simulink model "State_Flow_D"  (R2017a)
settings: Solver=FixedStepDiscrete  StartTime=0.0  StopTime=inf  FixedStep=0.001  RelTol=1e-3  EnableMultiTasking=on
libraries: xpcethercatlib x35, simulink x11, commutil2 x2
(part 1 of 3)
settings Model: SimulationMode=external  Creator=simoc  LastModifiedBy=Danie
settings SolverCC: EnableConcurrentExecution=on  ConcurrentTasks=on  AutoInsertRateTranBlk=on
settings DataIOCC: SaveFormat=StructureWithTime
settings OptimizationCC: BlockReduction=off  OptimizeBlockIOStorage=off  BufferReuse=off  GlobalBufferReuse=off  ExpressionFolding=off  LocalBlockOutputs=off
settings HardwareCC: ProdBitPerPointer=32  ProdBitPerSizeT=32  ProdBitPerPtrDiffT=32  ProdLargestAtomicFloat=None  ProdWordSize=32  ProdLongLongMode=on  ProdHWDeviceType=Generic->32-bit x86 compatible
settings RTWCC: SystemTargetFile=slrt.tlc  TemplateMakefile=slrt_default_tmf  Description=Simulink Real-Time  RTWCompilerOptimization=on
settings SimulinkRealTimeCC: xPCConcurrentTasks=on

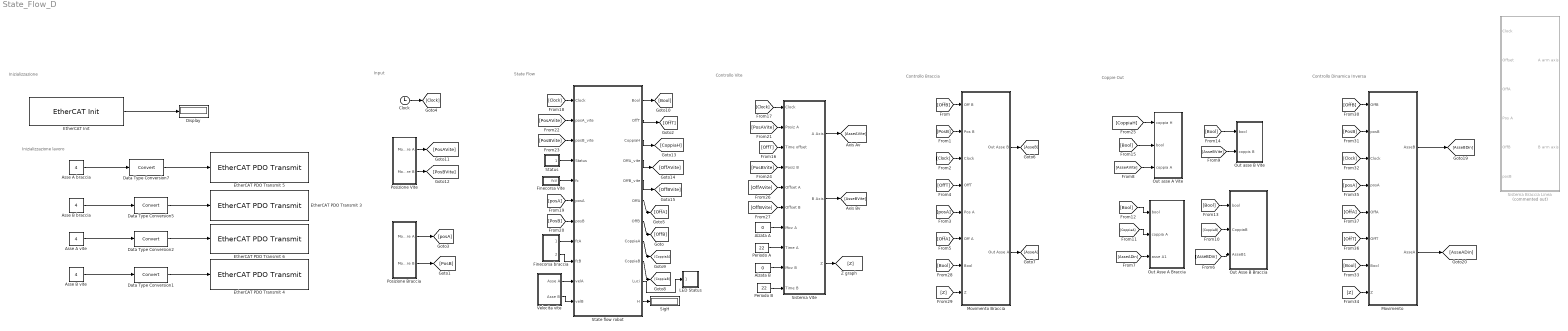
== system State_Flow_D ==
  note: Input
  note: State Flow
  note: Coppie Out
  note: Controllo Braccia
  note: Controllo Vite
  note: Inizializzazione
  note: Inizializzazione lavoro
  note: Controllo Dinamica Inversa
  Alzata A : Constant  Value=0
  "Alzata B " : Constant  Value=0
  Asse A braccia : Constant  Value=4
  Asse A vite : Constant  Value=4
  Asse B braccia : Constant  Value=4
  Asse B vite : Constant  Value=4
  Clock : Clock
  Data Type Conversion{1..2,5,7} (4 alike) : DataTypeConversion
  Display : Display
  "EtherCAT Init " : xpcethercatlib/EtherCAT Init   Priority=0  config_file=C:\Users\Danie\Documenti\Github\PKMRobot\final_net.xml  device_id=0  pci_bus=4  pci_slot=1  dctuning=0  enaDebug=off  enaDC=on  errLink=off  masterDbg=off  stateChgDbg=off  baseClock=off  masterCfg=off  logFile='c:\dbglog.txt'  sample_time=0.001000  DCMode=1
      settings: SourceProductName=Simulink Real-Time  SourceProductBaseCode=XP
  EtherCAT PDO Transmit 3 : xpcethercatlib/EtherCAT PDO Transmit   Priority=3  sig_name=AZ2.Receive PDO 1.Axis A Modes of operation  sig_offset=264  sig_type=int8  type_size=8  sig_dim=1  device_id=0  sample_time=0.001000
      settings: SourceProductName=Simulink Real-Time  SourceProductBaseCode=XP
  EtherCAT PDO Transmit 4 : xpcethercatlib/EtherCAT PDO Transmit   Priority=3  sig_name=AZ2.Receive PDO 1.Axis A Modes of operation  sig_offset=264  sig_type=int8  type_size=8  sig_dim=1  device_id=0  sample_time=0.001000
      settings: SourceProductName=Simulink Real-Time  SourceProductBaseCode=XP
  EtherCAT PDO Transmit 5 : xpcethercatlib/EtherCAT PDO Transmit   Priority=3  sig_name=AZ2.Receive PDO 2.Axis B Modes of operation  sig_offset=288  sig_type=int8  type_size=8  sig_dim=1  device_id=0  sample_time=0.001000
      settings: SourceProductName=Simulink Real-Time  SourceProductBaseCode=XP
  EtherCAT PDO Transmit 6 : xpcethercatlib/EtherCAT PDO Transmit   Priority=3  sig_name=AZ2.Receive PDO 1.Axis A Modes of operation  sig_offset=264  sig_type=int8  type_size=8  sig_dim=1  device_id=0  sample_time=0.001000
      settings: SourceProductName=Simulink Real-Time  SourceProductBaseCode=XP
  Finecorsa Vite : Subsystem
  Finecorsa braccia : Subsystem
  LED Status : Subsystem
  Movimento : Subsystem
  Movimento Braccia : Subsystem
  Out Asse A Braccia : Subsystem
  Out Asse B Braccia : Subsystem
  Out asse A Vite : Subsystem
  Out asse B Vite : Subsystem
  Periodo A : Constant  Value=22
  Periodo B : Constant  Value=22
  "Posizione Braccia " : Subsystem
  Posizione Vite : Subsystem
  SigH : Display
  Sistema Braccia Linea : Subsystem  Commented=on
  Sistema Vite : Subsystem
  State flow robot : Stateflow chart  TreatAsAtomicUnit=on
  Status : Subsystem
  "Velocita vite " : Subsystem
  wires:
  "EtherCAT Init "/1 -> Display/1
  Data Type Conversion7/1 -> EtherCAT PDO Transmit 5/1
  Asse A braccia/1 -> Data Type Conversion7/1
  Data Type Conversion5/1 -> EtherCAT PDO Transmit 3/1
  Asse B braccia/1 -> Data Type Conversion5/1
  Clock/1 -> [Clock]
  State flow robot/1(Bool) -> [Bool]
  Data Type Conversion1/1 -> EtherCAT PDO Transmit 4/1
  Asse B vite/1 -> Data Type Conversion1/1
  Data Type Conversion2/1 -> EtherCAT PDO Transmit 6/1
  Asse A vite/1 -> Data Type Conversion2/1
  Posizione Vite/2(Motore B) -> [PosBVite]
  Status/1(Word) -> State flow robot/4(Status)
  State flow robot/2(OffT) -> [OffT]
  Alzata A/1 -> Sistema Vite/7(Mov A)
  Periodo A/1 -> Sistema Vite/8(Time A)
  "Alzata B "/1 -> Sistema Vite/9(Mov B)
  Periodo B/1 -> Sistema Vite/10(Time B)
  Finecorsa Vite/1(fcV) -> State flow robot/5(fc)
  Finecorsa braccia/1(Asse A) -> State flow robot/8(fcA)
  Finecorsa braccia/2(Asse B) -> State flow robot/9(fcB)
  "Posizione Braccia "/2(Motore B) -> [PosB]
  "Posizione Braccia "/1(Motore A) -> [posA]
  Posizione Vite/1(Motore A) -> [PosAVite]
  State flow robot/10(Luci) -> LED Status/1(Luci)
  "Velocita vite "/1(Asse A) -> State flow robot/10(velA)
  "Velocita vite "/2(Asse B) -> State flow robot/11(velB)
  State flow robot/7(OffB) -> [OffB]
  State flow robot/6(OffA) -> [OffA]
  [AsseBDin] -> Out Asse B Braccia/3(AsseB1)
  [AsseADin] -> Out Asse A Braccia/3(asse A1)
  [CoppiaB] -> Out Asse B Braccia/2(CoppiaB)
  State flow robot/9(CoppiaB) -> [CoppiaB]
  State flow robot/8(CoppiaA) -> [CoppiaA]
  [CoppiaA] -> Out Asse A Braccia/2(coppia A)
  [Bool] -> Out Asse A Braccia/1(bool)
  [Bool] -> Out Asse B Braccia/1(bool)
  [Bool] -> Out asse B Vite/1(bool)
  [Bool] -> Out asse A Vite/2(bool)
  [OffT] -> Sistema Vite/3(Time offset)
  [Clock] -> Sistema Vite/1(Clock)
  [Clock] -> State flow robot/1(Clock)
  [posA] -> State flow robot/6(posA)
  [PosB] -> State flow robot/7(posB)
  [PosAVite] -> Sistema Vite/2(Posiz A)
  [PosAVite] -> State flow robot/2(posA_vite)
  [PosBVite] -> State flow robot/3(posB_vite)
  [PosBVite] -> Sistema Vite/4(Posiz B)
  State flow robot/3(CoppiaH) -> [CoppiaH]
  [CoppiaH] -> Out asse A Vite/1(coppia H)
  State flow robot/4(OffA_vite) -> [OffAVite]
  [OffAVite] -> Sistema Vite/5(Offset A)
  State flow robot/5(OffB_vite) -> [OffBVite]
  [OffBVite] -> Sistema Vite/6(Offset B)
  [OffB] -> Movimento Braccia/1(Off B)
  [PosB] -> Movimento Braccia/2(Pos B)
  [Clock] -> Movimento Braccia/3(Clock)
  [OffT] -> Movimento Braccia/4(OffT)
  [posA] -> Movimento Braccia/5(Pos A)
  [OffA] -> Movimento Braccia/6(Off A)
  Movimento Braccia/1(Out Asse B) -> [AsseB]
  Movimento Braccia/2(Out Asse A) -> [AsseA]
  Sistema Vite/1(A Axis) -> [AsseAVite]
  [AsseAVite] -> Out asse A Vite/3(coppia A)
  Sistema Vite/2(B Axis) -> [AsseBVite]
  [AsseBVite] -> Out asse B Vite/2(coppis B)
  [Bool] -> Movimento Braccia/7("Bool ")
  Sistema Vite/3(Z) -> [Z]
  [Z] -> Movimento Braccia/8(Z)
  [PosB] -> Movimento/2(posB)
  Movimento/2(AsseA) -> [AsseADin]
  Movimento/1(AsseB) -> [AsseBDin]
  [OffA] -> Movimento/5(OffA)
  [OffT] -> Movimento/6(OffT)
  [OffB] -> Movimento/1(OffB)
  [Clock] -> Movimento/3(Clock)
  [posA] -> Movimento/4(posA)
  [Bool] -> Movimento/7("Bool ")
  [Z] -> Movimento/8(Z)
  State flow robot/11(H) -> SigH/1

== system State_Flow_D/Finecorsa Vite ==
  Data Type Conversion8 : DataTypeConversion
  EtherCAT PDO Receive16 : xpcethercatlib/EtherCAT PDO Receive  Priority=2  sig_name=AZ2.Transmit PDO 3.General purpose inputs  sig_offset=440  sig_type=uint16  type_size=16  sig_dim=1  device_id=0  sample_time=0.001000
      settings: SourceProductName=Simulink Real-Time  SourceProductBaseCode=XP
  Integer to Bit Converter : commutil2/Integer to Bit Converter  nbits=16  signedInputValues=Unsigned  bitOrder=LSB first  outDtype=Inherit via internal rule
  Selector : Selector  InputPortWidth=16  IndexOptions=Index vector (dialog)  Indices=15  OutputSizes=1
  fcV : Outport
  wires:
  EtherCAT PDO Receive16/1 -> Data Type Conversion8/1
  Selector/1 -> fcV/1
  Data Type Conversion8/1 -> Integer to Bit Converter/1
  Integer to Bit Converter/1 -> Selector/1

== system State_Flow_D/Finecorsa braccia ==
  Data Type Conversion8 : DataTypeConversion
  EtherCAT PDO Receive16 : xpcethercatlib/EtherCAT PDO Receive  Priority=2  sig_name=AZ1.Transmit PDO 3.General purpose inputs  sig_offset=184  sig_type=uint16  type_size=16  sig_dim=1  device_id=0  sample_time=0.001000
      settings: SourceProductName=Simulink Real-Time  SourceProductBaseCode=XP
  Integer to Bit Converter : commutil2/Integer to Bit Converter  nbits=16  signedInputValues=Unsigned  bitOrder=LSB first  outDtype=Inherit via internal rule
  Selector : Selector  InputPortWidth=16  IndexOptions=Index vector (dialog)  Indices=8  OutputSizes=1
  Selector1 : Selector  InputPortWidth=16  IndexOptions=Index vector (dialog)  Indices=15  OutputSizes=1
  Asse A : Outport
  Asse B : Outport  Port=2
  wires:
  Data Type Conversion8/1 -> Integer to Bit Converter/1
  Integer to Bit Converter/1 -> Selector1/1, Selector/1
  EtherCAT PDO Receive16/1 -> Data Type Conversion8/1
  Selector1/1 -> Asse B/1
  Selector/1 -> Asse A/1

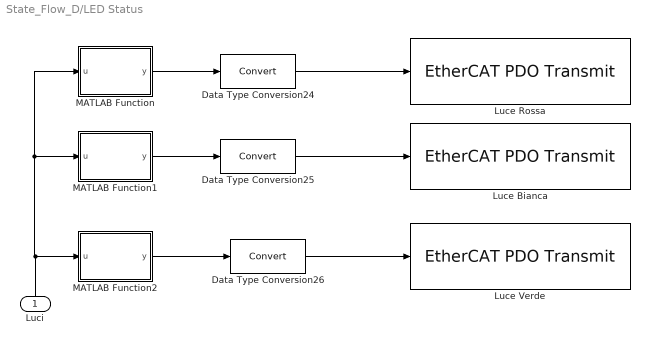
== system State_Flow_D/LED Status ==
  Luci : Inport
  Data Type Conversion24 : DataTypeConversion
  Data Type Conversion25 : DataTypeConversion
  Data Type Conversion26 : DataTypeConversion
  Luce Bianca : xpcethercatlib/EtherCAT PDO Transmit   Priority=3  sig_name=Beckoff.Channel 6.Output  sig_offset=1  sig_type=boolean  type_size=1  sig_dim=1  device_id=0  sample_time=0.001000
      settings: SourceProductName=Simulink Real-Time  SourceProductBaseCode=XP
  "Luce Rossa " : xpcethercatlib/EtherCAT PDO Transmit   Priority=3  sig_name=Beckoff.Channel 8.Output  sig_offset=3  sig_type=boolean  type_size=1  sig_dim=1  device_id=0  sample_time=0.001000
      settings: SourceProductName=Simulink Real-Time  SourceProductBaseCode=XP
  Luce Verde : xpcethercatlib/EtherCAT PDO Transmit   Priority=3  sig_name=Beckoff.Channel 7.Output  sig_offset=2  sig_type=boolean  type_size=1  sig_dim=1  device_id=0  sample_time=0.001000
      settings: SourceProductName=Simulink Real-Time  SourceProductBaseCode=XP
  MATLAB Function : MATLAB Function  TreatAsAtomicUnit=on
  MATLAB Function1 : MATLAB Function  TreatAsAtomicUnit=on
  MATLAB Function2 : MATLAB Function  TreatAsAtomicUnit=on
  wires:
  MATLAB Function2/1(y) -> Data Type Conversion26/1
  MATLAB Function/1(y) -> Data Type Conversion24/1
  Data Type Conversion26/1 -> Luce Verde/1
  MATLAB Function1/1(y) -> Data Type Conversion25/1
  Data Type Conversion24/1 -> "Luce Rossa "/1
  Data Type Conversion25/1 -> Luce Bianca/1
  Luci/1 -> MATLAB Function/1(u), MATLAB Function1/1(u), MATLAB Function2/1(u)

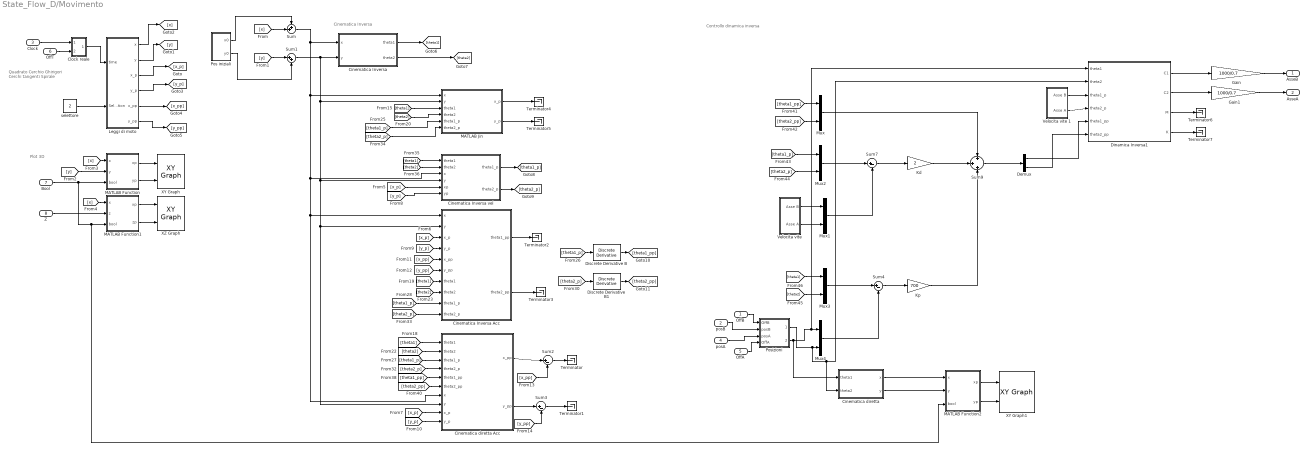
== system State_Flow_D/Movimento ==
  note: Cinematica Inversa
  note: Controllo dinamica inversa
  note: Plot 3D
  note: Quadrato
      | Cerchio
      | Ghirigori
      | Cerchi tangenti
      | Spirale
  OffB : Inport
  posB : Inport  Port=2
  Clock : Inport  Port=3
  posA : Inport  Port=4
  OffA : Inport  Port=5
  OffT : Inport  Port=6
  "Bool " : Inport  Port=7
  Z : Inport  Port=8
  Cinematica Inversa : MATLAB Function  TreatAsAtomicUnit=on
  Cinematica Inversa Acc : MATLAB Function  TreatAsAtomicUnit=on
  Cinematica Inversa vel : MATLAB Function  TreatAsAtomicUnit=on
  Cinematica diretta : MATLAB Function  TreatAsAtomicUnit=on
  Cinematica diretta Acc : MATLAB Function  TreatAsAtomicUnit=on
  Clock reale : Subsystem
  Demux : Demux  Outputs=2
  Dinamica Inversa1 : MATLAB Function  TreatAsAtomicUnit=on
  Discrete Derivative B : simulink/Discrete/Discrete Derivative  gainval=1.0  ICPrevScaledInput=0.0  OutMin=[]  OutMax=[]  OutDataType=fixdt(1, 16)  OutScaling=2^-10  DoSatur=off
  Discrete Derivative B1 : simulink/Discrete/Discrete Derivative  gainval=1.0  ICPrevScaledInput=0.0  OutMin=[]  OutMax=[]  OutDataType=fixdt(1, 16)  OutScaling=2^-10  DoSatur=off
  Gain : Gain  Gain=1000/0.7
  Gain1 : Gain  Gain=1000/0.7
  Kd : Gain  Gain=2
  Kp : Gain  Gain=700
  Leggi di moto : Subsystem
  MATLAB Function : MATLAB Function  TreatAsAtomicUnit=on
  MATLAB Function1 : MATLAB Function  TreatAsAtomicUnit=on
  MATLAB Function2 : MATLAB Function  TreatAsAtomicUnit=on
  MATLAB Jin : MATLAB Function  TreatAsAtomicUnit=on
  Mux{,1..4} (5 alike) : Mux  Inputs=2
  Pos iniziali : Subsystem
  Posizioni : Subsystem
  Sum : Sum  Inputs=++|
  Sum1 : Sum  Inputs=|++
  Sum{2..4,7} (4 alike) : Sum  Inputs=|+-
  Sum9 : Sum  Inputs=+|+|+
  Terminator{,1..7} (8 alike) : Terminator
  "Velocita vite " : Subsystem
  Velocita vite 1 : Subsystem
  XY Graph : simulink/Sinks/XY Graph  xmin=-0.1  xmax=0.1  ymin=-0.1  ymax=0.1  st=0.001
  XY Graph1 : simulink/Sinks/XY Graph  xmin=-0.15  xmax=0.15  ymin=0  ymax=0.5  st=0.001
  XZ Graph : simulink/Sinks/XY Graph  xmin=-0.15  xmax=0.15  ymin=-0.15  ymax=0.15  st=0.001
  selettore : Constant  Value=2
  AsseB : Outport
  AsseA : Outport  Port=2
  wires:
  Sum/1 -> Cinematica diretta Acc/7(x), Cinematica Inversa Acc/1(x), Cinematica Inversa vel/3(x), MATLAB Jin/1(x), Cinematica Inversa/1(x)
  Clock/1 -> Clock reale/1(cr)
  OffT/1 -> Clock reale/2(offset)
  Cinematica diretta Acc/1(x_pp) -> Sum2/1
  Cinematica diretta Acc/2(y_pp) -> Sum3/1
  Sum2/1 -> Terminator/1
  Sum3/1 -> Terminator1/1
  MATLAB Jin/1(x_p) -> Terminator4/1
  MATLAB Jin/2(y_p) -> Terminator5/1
  Sum1/1 -> Cinematica diretta Acc/8(y), Cinematica Inversa Acc/2(y), Cinematica Inversa vel/4(y), MATLAB Jin/2(y), Cinematica Inversa/2(y)
  Clock reale/1(Ck) -> Leggi di moto/1(time)
  Leggi di moto/2(y) -> [y]
  [x] -> MATLAB Function1/1(x)
  [x] -> MATLAB Function/1(x)
  Leggi di moto/1(x) -> [x]
  Leggi di moto/3(x_p) -> [x_p]
  [y] -> MATLAB Function/2(y)
  selettore/1 -> Leggi di moto/2(Selection)
  MATLAB Function/1(xp) -> XY Graph/1
  MATLAB Function1/1(xp) -> XZ Graph/1
  Z/1 -> MATLAB Function1/2(z)
  Leggi di moto/4(y_p) -> [y_p]
  MATLAB Function1/2(zp) -> XZ Graph/2
  MATLAB Function/2(yp) -> XY Graph/2
  [y] -> Sum1/1
  Leggi di moto/5(x_pp) -> [x_pp]
  Leggi di moto/6(y_pp) -> [y_pp]
  [x_p] -> Cinematica Inversa vel/5(xp)
  [x_p] -> Cinematica Inversa Acc/3(x_p)
  [x_p] -> Cinematica diretta Acc/9(x_p)
  [y_p] -> Cinematica Inversa vel/6(yp)
  [y_p] -> Cinematica Inversa Acc/4(y_p)
  [y_p] -> Cinematica diretta Acc/10(y_p)
  [x_pp] -> Cinematica Inversa Acc/5(x_pp)
  [y_pp] -> Cinematica Inversa Acc/6(y_pp)
  [x_pp] -> Sum2/2
  [y_pp] -> Sum3/2
  Cinematica Inversa Acc/1(theta1_pp) -> Terminator2/1
  Cinematica Inversa Acc/2(theta2_pp) -> Terminator3/1
  OffB/1 -> Posizioni/1(OffB)
  posB/1 -> Posizioni/2(posB)
  posA/1 -> Posizioni/3(posA)
  OffA/1 -> Posizioni/4(OffA)
  Cinematica Inversa/1(theta1) -> [theta1]
  [theta1] -> MATLAB Jin/3(theta1)
  [theta1] -> Cinematica diretta Acc/1(theta1)
  [theta1] -> Cinematica Inversa Acc/7(theta1)
  Cinematica Inversa/2(theta2) -> [theta2]
  [theta2] -> MATLAB Jin/4(theta2)
  [theta2] -> Cinematica diretta Acc/2(theta2)
  [theta2] -> Cinematica Inversa Acc/8(theta2)
  Cinematica Inversa vel/1(theta1_p) -> [theta1_p]
  [theta1_p] -> MATLAB Jin/5(theta1_p)
  [theta1_p] -> Discrete Derivative B/1
  [theta1_p] -> Cinematica diretta Acc/3(theta1_p)
  [theta1_p] -> Cinematica Inversa Acc/9(theta1_p)
  Cinematica Inversa vel/2(theta2_p) -> [theta2_p]
  [theta2_p] -> Discrete Derivative B1/1
  [theta2_p] -> Cinematica diretta Acc/4(theta2_p)
  [theta2_p] -> Cinematica Inversa Acc/10(theta2_p)
  [theta2_p] -> MATLAB Jin/6(theta2_p)
  [theta1] -> Cinematica Inversa vel/1(theta1)
  [theta2] -> Cinematica Inversa vel/2(theta2)
  Discrete Derivative B/1 -> [theta1_pp]
  [theta1_pp] -> Cinematica diretta Acc/5(theta1_pp)
  Discrete Derivative B1/1 -> [theta2_pp]
  [theta2_pp] -> Cinematica diretta Acc/6(theta2_pp)
  Pos iniziali/2(y0) -> Sum1/2
  [x] -> Sum/2
  Pos iniziali/1(x0) -> Sum/1
  [theta1_pp] -> Mux/1
  [theta2_pp] -> Mux/2
  "Velocita vite "/2(Asse A) -> Mux1/2
  "Velocita vite "/1(Asse B) -> Mux1/1
  [theta1_p] -> Mux2/1
  [theta2_p] -> Mux2/2
  [theta1] -> Mux3/1
  [theta2] -> Mux3/2
  Mux2/1 -> Sum7/1
  Mux1/1 -> Sum7/2
  Mux3/1 -> Sum4/1
  Mux4/1 -> Sum4/2
  Mux/1 -> Sum9/1
  Sum7/1 -> Kd/1
  Sum4/1 -> Kp/1
  Kp/1 -> Sum9/3
  Kd/1 -> Sum9/2
  Sum9/1 -> Demux/1
  Velocita vite 1/2(Asse A) -> Dinamica Inversa1/4(theta2_p)
  Velocita vite 1/1(Asse B) -> Dinamica Inversa1/3(theta1_p)
  Posizioni/2(Asse Bb) -> Cinematica diretta/1(theta1), Dinamica Inversa1/1(theta1), Mux4/1
  Posizioni/1(Asse Ab) -> Cinematica diretta/2(theta2), Dinamica Inversa1/2(theta2), Mux4/2
  Demux/1 -> Dinamica Inversa1/5(theta1_pp)
  Demux/2 -> Dinamica Inversa1/6(theta2_pp)
  Dinamica Inversa1/1(C1) -> Gain/1
  Dinamica Inversa1/2(C2) -> Gain1/1
  Gain/1 -> AsseB/1
  Gain1/1 -> AsseA/1
  MATLAB Function2/1(xp) -> XY Graph1/1
  MATLAB Function2/2(yp) -> XY Graph1/2
  "Bool "/1 -> MATLAB Function2/3(bool), MATLAB Function1/3(bool), MATLAB Function/3(bool)
  Cinematica diretta/2(y) -> MATLAB Function2/2(y)
  Cinematica diretta/1(x) -> MATLAB Function2/1(x)
  Dinamica Inversa1/3(M) -> Terminator6/1
  Dinamica Inversa1/4(K) -> Terminator7/1

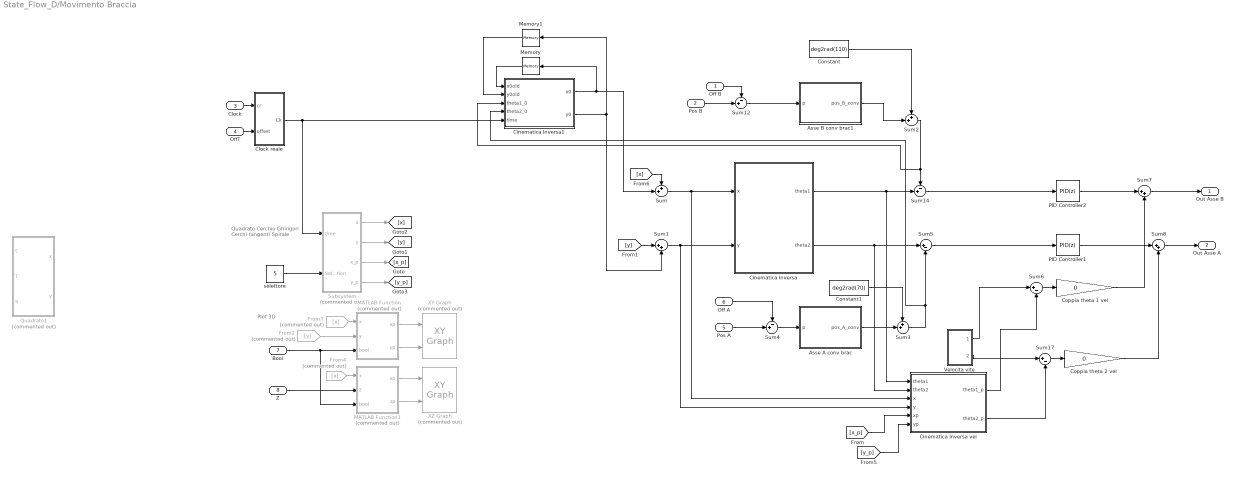
== system State_Flow_D/Movimento Braccia ==
  note: Plot 3D
  note: Quadrato
      | Cerchio
      | Ghirigori
      | Cerchi tangenti
      | Spirale
  Off B : Inport
  Pos B : Inport  Port=2
  Clock : Inport  Port=3
  OffT : Inport  Port=4
  Pos A : Inport  Port=5
  Off A : Inport  Port=6
  "Bool " : Inport  Port=7
  Z : Inport  Port=8
  Asse A conv brac : MATLAB Function  TreatAsAtomicUnit=on
  Asse B conv brac1 : MATLAB Function  TreatAsAtomicUnit=on
  Cinematica Inversa : MATLAB Function  TreatAsAtomicUnit=on
  Cinematica Inversa vel : MATLAB Function  TreatAsAtomicUnit=on
  Cinematica Inversa1 : MATLAB Function  TreatAsAtomicUnit=on
  Clock reale : Subsystem
  Constant : Constant  Value=deg2rad(110)
  Constant1 : Constant  Value=deg2rad(70)
  Coppia theta 1 vel : Gain  Gain=0
  Coppia theta 2 vel : Gain  Gain=0
  From2 : From  Commented=on  GotoTag=y
  From3 : From  Commented=on  GotoTag=x
  From4 : From  Commented=on  GotoTag=x
  MATLAB Function : MATLAB Function  Commented=on  TreatAsAtomicUnit=on
  MATLAB Function1 : MATLAB Function  Commented=on  TreatAsAtomicUnit=on
  Memory : Memory
  Memory1 : Memory
  PID Controller1 : simulink/Continuous/PID Controller  Controller=PID  TimeDomain=Discrete-time  SampleTime=-1  IntegratorMethod=Forward Euler  FilterMethod=Forward Euler  Form=Parallel  UseFilter=on  ControllerParametersSource=internal  P=3e+05  I=100  D=0  N=100  InitialConditionSource=internal  InitialConditionForIntegrator=0  InitialConditionForFilter=0  ExternalReset=none  LimitOutput=off  UpperSaturationLimit=inf  LowerSaturationLimit=-inf  LinearizeAsGain=on  AntiWindupMode=none  Kb=1  TrackingMode=off  Kt=1  PParamMin=[]  PParamMax=[]  IParamMin=[]  IParamMax=[]  DParamMin=[]  DParamMax=[]  NParamMin=[]  NParamMax=[]  KbParamMin=[]  KbParamMax=[]  KtParamMin=[]  KtParamMax=[]  POutMin=[]  POutMax=[]  IOutMin=[]  IOutMax=[]  DOutMin=[]  DOutMax=[]  NOutMin=[]  NOutMax=[]  KbOutMin=[]  KbOutMax=[]  KtOutMin=[]  KtOutMax=[]  IntegratorOutMin=[]  IntegratorOutMax=[]  FilterOutMin=[]  FilterOutMax=[]  SumOutMin=[]  SumOutMax=[]  SumI1OutMin=[]  SumI1OutMax=[]  SumI2OutMin=[]  SumI2OutMax=[]  SumI3OutMin=[]  SumI3OutMax=[]  SumDOutMin=[]  SumDOutMax=[]  SaturationOutMin=[]  SaturationOutMax=[]  IntegratorContinuousStateAttributes=''  IntegratorStateMustResolveToSignalObject=off  IntegratorRTWStateStorageClass=Auto  FilterContinuousStateAttributes=''  FilterStateMustResolveToSignalObject=off  FilterRTWStateStorageClass=Auto  DifferentiatorICPrevScaledInput=0  DifferentiatorOutMin=[]  DifferentiatorOutMax=[]  InitialConditionSetting=State (most efficient)
  PID Controller2 : simulink/Continuous/PID Controller  Controller=PID  TimeDomain=Discrete-time  SampleTime=-1  IntegratorMethod=Forward Euler  FilterMethod=Forward Euler  Form=Parallel  UseFilter=on  ControllerParametersSource=internal  P=3e+05  I=100  D=0  N=100  InitialConditionSource=internal  InitialConditionForIntegrator=0  InitialConditionForFilter=0  ExternalReset=none  LimitOutput=off  UpperSaturationLimit=inf  LowerSaturationLimit=-inf  LinearizeAsGain=on  AntiWindupMode=none  Kb=1  TrackingMode=off  Kt=1  PParamMin=[]  PParamMax=[]  IParamMin=[]  IParamMax=[]  DParamMin=[]  DParamMax=[]  NParamMin=[]  NParamMax=[]  KbParamMin=[]  KbParamMax=[]  KtParamMin=[]  KtParamMax=[]  POutMin=[]  POutMax=[]  IOutMin=[]  IOutMax=[]  DOutMin=[]  DOutMax=[]  NOutMin=[]  NOutMax=[]  KbOutMin=[]  KbOutMax=[]  KtOutMin=[]  KtOutMax=[]  IntegratorOutMin=[]  IntegratorOutMax=[]  FilterOutMin=[]  FilterOutMax=[]  SumOutMin=[]  SumOutMax=[]  SumI1OutMin=[]  SumI1OutMax=[]  SumI2OutMin=[]  SumI2OutMax=[]  SumI3OutMin=[]  SumI3OutMax=[]  SumDOutMin=[]  SumDOutMax=[]  SaturationOutMin=[]  SaturationOutMax=[]  IntegratorContinuousStateAttributes=''  IntegratorStateMustResolveToSignalObject=off  IntegratorRTWStateStorageClass=Auto  FilterContinuousStateAttributes=''  FilterStateMustResolveToSignalObject=off  FilterRTWStateStorageClass=Auto  DifferentiatorICPrevScaledInput=0  DifferentiatorOutMin=[]  DifferentiatorOutMax=[]  InitialConditionSetting=State (most efficient)
  Quadrato1 : MATLAB Function  Commented=on  TreatAsAtomicUnit=on
  Subsystem : Subsystem  Commented=on
  Sum : Sum  Inputs=++|
  Sum1 : Sum  Inputs=|++
  Sum12 : Sum  Inputs=-+|
  Sum14 : Sum  Inputs=-+|
  Sum17 : Sum  Inputs=|+-
  Sum2 : Sum  Inputs=++|
  Sum3 : Sum  Inputs=++|
  Sum4 : Sum  Inputs=-+|
  Sum5 : Sum  Inputs=|+-
  Sum6 : Sum  Inputs=|+-
  Sum7 : Sum  Inputs=|++
  Sum8 : Sum  Inputs=|++
  "Velocita vite " : Subsystem
  XY Graph : simulink/Sinks/XY Graph  Commented=on  xmin=-0.1  xmax=0.1  ymin=-0.1  ymax=0.1  st=0.001
  XZ Graph : simulink/Sinks/XY Graph  Commented=on  xmin=-0.15  xmax=0.15  ymin=-0.15  ymax=0.15  st=0.001
  selettore : Constant  Value=5
  Out Asse B : Outport
  Out Asse A : Outport  Port=2
  wires:
  Off A/1 -> Sum4/1
  Asse A conv brac/1(pos_A_conv) -> Sum3/2
  Sum5/1 -> PID Controller1/1
  Cinematica Inversa1/2(y0) -> Memory1/1, Sum1/2
  Sum/1 -> Cinematica Inversa vel/3(x), Cinematica Inversa/1(x)
  Constant1/1 -> Sum3/1
  Constant/1 -> Sum2/1
  Sum1/1 -> Cinematica Inversa vel/4(y), Cinematica Inversa/2(y)
  Sum4/1 -> Asse A conv brac/1(p)
  Pos A/1 -> Sum4/2
  Sum12/1 -> Asse B conv brac1/1(p)
  Pos B/1 -> Sum12/2
  Sum14/1 -> PID Controller2/1
  Off B/1 -> Sum12/1
  Clock/1 -> Clock reale/1(cr)
  OffT/1 -> Clock reale/2(offset)
  Sum6/1 -> Coppia theta 1 vel/1
  "Velocita vite "/1(Asse B) -> Sum6/1
  Sum17/1 -> Coppia theta 2 vel/1
  Cinematica Inversa vel/1(theta1_p) -> Sum6/2
  PID Controller2/1 -> Sum7/1
  Coppia theta 1 vel/1 -> Sum7/2
  Sum7/1 -> Out Asse B/1
  PID Controller1/1 -> Sum8/1
  Sum8/1 -> Out Asse A/1
  Coppia theta 2 vel/1 -> Sum8/2
  Cinematica Inversa1/1(x0) -> Sum/2, Memory/1
  Memory1/1 -> Cinematica Inversa1/2(y0old)
  Memory/1 -> Cinematica Inversa1/1(x0old)
  Cinematica Inversa/1(theta1) -> Cinematica Inversa vel/1(theta1), Sum14/2
  Sum2/1 -> Cinematica Inversa1/3(theta1_0), Sum14/1
  Cinematica Inversa/2(theta2) -> Cinematica Inversa vel/2(theta2), Sum5/1
  Clock reale/1(Ck) -> Subsystem/1(time), Cinematica Inversa1/5(time)
  Sum3/1 -> Cinematica Inversa1/4(theta2_0), Sum5/2
  "Bool "/1 -> MATLAB Function1/3(bool), MATLAB Function/3(bool)
  MATLAB Function/1(xp) -> XY Graph/1
  MATLAB Function/2(yp) -> XY Graph/2
  Z/1 -> MATLAB Function1/2(z)
  MATLAB Function1/2(zp) -> XZ Graph/2
  MATLAB Function1/1(xp) -> XZ Graph/1
  selettore/1 -> Subsystem/2(Selection)
  Subsystem/3(x_p) -> [x_p]
  [x_p] -> Cinematica Inversa vel/5(xp)
  Subsystem/2(y) -> [y]
  Subsystem/1(x) -> [x]
  Subsystem/4(y_p) -> [y_p]
  [y] -> Sum1/1
  From2/1 -> MATLAB Function/2(y)
  From3/1 -> MATLAB Function/1(x)
  From4/1 -> MATLAB Function1/1(x)
  [y_p] -> Cinematica Inversa vel/6(yp)
  [x] -> Sum/1
  Asse B conv brac1/1(pos_B_conv) -> Sum2/2
  "Velocita vite "/2(Asse A) -> Sum17/1
  Cinematica Inversa vel/2(theta2_p) -> Sum17/2

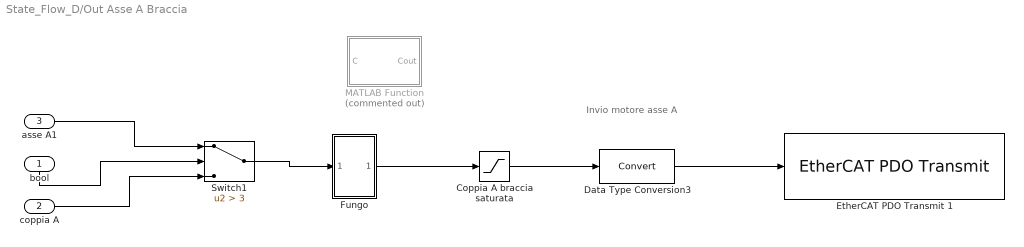
== system State_Flow_D/Out Asse A Braccia ==
  note: Invio motore asse A
  bool : Inport
  coppia A : Inport  Port=2
  asse A1 : Inport  Port=3
  Coppia A braccia saturata : Saturate  UpperLimit=2500  LowerLimit=-2500
  Data Type Conversion3 : DataTypeConversion
  EtherCAT PDO Transmit 1 : xpcethercatlib/EtherCAT PDO Transmit   Priority=3  sig_name=AZ1.Receive PDO 1.Axis A Target Torque  sig_offset=16  sig_type=int16  type_size=16  sig_dim=1  device_id=0  sample_time=0.001000
      settings: SourceProductName=Simulink Real-Time  SourceProductBaseCode=XP
  Fungo : Subsystem
  MATLAB Function : MATLAB Function  Commented=on  TreatAsAtomicUnit=on
  Switch1 : Switch  Criteria=u2 > Threshold  Threshold=3
  wires:
  Data Type Conversion3/1 -> EtherCAT PDO Transmit 1/1
  bool/1 -> Switch1/2
  asse A1/1 -> Switch1/1
  coppia A/1 -> Switch1/3
  Switch1/1 -> Fungo/1(In1)
  Coppia A braccia saturata/1 -> Data Type Conversion3/1
  Fungo/1(Out1) -> Coppia A braccia saturata/1

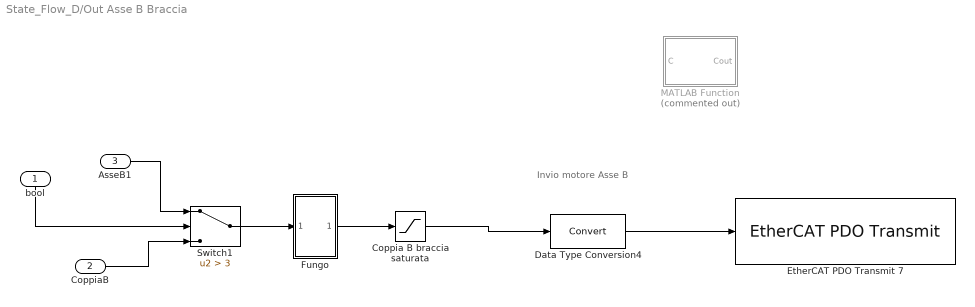
== system State_Flow_D/Out Asse B Braccia ==
  note: Invio motore Asse B
  bool : Inport
  CoppiaB : Inport  Port=2
  AsseB1 : Inport  Port=3
  Coppia B braccia saturata : Saturate  UpperLimit=2500  LowerLimit=-2500
  Data Type Conversion4 : DataTypeConversion
  EtherCAT PDO Transmit 7 : xpcethercatlib/EtherCAT PDO Transmit   Priority=3  sig_name=AZ1.Receive PDO 2.Axis B Target Torque  sig_offset=40  sig_type=int16  type_size=16  sig_dim=1  device_id=0  sample_time=0.001000
      settings: SourceProductName=Simulink Real-Time  SourceProductBaseCode=XP
  Fungo : Subsystem
  MATLAB Function : MATLAB Function  Commented=on  TreatAsAtomicUnit=on
  Switch1 : Switch  Criteria=u2 > Threshold  Threshold=3
  wires:
  Data Type Conversion4/1 -> EtherCAT PDO Transmit 7/1
  AsseB1/1 -> Switch1/1
  Switch1/1 -> Fungo/1(In1)
  CoppiaB/1 -> Switch1/3
  bool/1 -> Switch1/2
  Fungo/1(Out1) -> Coppia B braccia saturata/1
  Coppia B braccia saturata/1 -> Data Type Conversion4/1

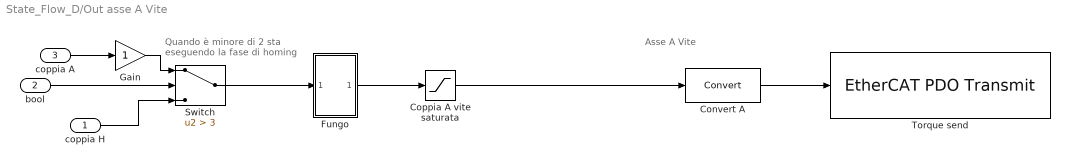
== system State_Flow_D/Out asse A Vite ==
  note: Quando è minore di 2 sta
      |  eseguendo la fase di homing
  note: Asse A Vite
  coppia H : Inport
  bool : Inport  Port=2
  coppia A : Inport  Port=3
  Convert A : DataTypeConversion
  Coppia A vite saturata : Saturate  UpperLimit=600  LowerLimit=-600
  Fungo : Subsystem
  Gain : Gain
  Switch : Switch  Criteria=u2 > Threshold  Threshold=3
  Torque send : xpcethercatlib/EtherCAT PDO Transmit   Priority=3  sig_name=AZ2.Receive PDO 1.Axis A Target Torque  sig_offset=272  sig_type=int16  type_size=16  sig_dim=1  device_id=0  sample_time=0.001000
      settings: SourceProductName=Simulink Real-Time  SourceProductBaseCode=XP
  wires:
  bool/1 -> Switch/2
  Convert A/1 -> Torque send/1
  coppia H/1 -> Switch/3
  coppia A/1 -> Gain/1
  Gain/1 -> Switch/1
  Switch/1 -> Fungo/1(In1)
  Coppia A vite saturata/1 -> Convert A/1
  Fungo/1(Out1) -> Coppia A vite saturata/1

== system State_Flow_D/Out asse B Vite ==
  note: Asse B Vite
  bool : Inport
  coppis B : Inport  Port=2
  Constant1 : Constant  Value=0
  Convert B : DataTypeConversion
  EtherCAT PDO Transmit 2 : xpcethercatlib/EtherCAT PDO Transmit   Priority=3  sig_name=AZ2.Receive PDO 2.Axis B Target Torque  sig_offset=296  sig_type=int16  type_size=16  sig_dim=1  device_id=0  sample_time=0.001000
      settings: SourceProductName=Simulink Real-Time  SourceProductBaseCode=XP
  Fungo : Subsystem
  Switch2 : Switch  Criteria=u2 > Threshold  Threshold=6
  wires:
  bool/1 -> Switch2/2
  coppis B/1 -> Switch2/1
  Constant1/1 -> Switch2/3
  Convert B/1 -> EtherCAT PDO Transmit 2/1
  Switch2/1 -> Fungo/1(In1)
  Fungo/1(Out1) -> Convert B/1

== system State_Flow_D/Posizione Braccia  ==
  Motore braccia A : xpcethercatlib/EtherCAT PDO Receive  Priority=2  sig_name=AZ1.Transmit PDO 1.Axis A Actual motor position  sig_offset=16  sig_type=int32  type_size=32  sig_dim=1  device_id=0  sample_time=0.001000
      settings: SourceProductName=Simulink Real-Time  SourceProductBaseCode=XP
  Motore braccia B : xpcethercatlib/EtherCAT PDO Receive  Priority=2  sig_name=AZ1.Transmit PDO 2.Axis B Actual motor position  sig_offset=104  sig_type=int32  type_size=32  sig_dim=1  device_id=0  sample_time=0.001000
      settings: SourceProductName=Simulink Real-Time  SourceProductBaseCode=XP
  convert : DataTypeConversion
  "convert 10 " : DataTypeConversion
  Motore A : Outport
  Motore B : Outport  Port=2
  wires:
  Motore braccia B/1 -> "convert 10 "/1
  Motore braccia A/1 -> convert/1
  "convert 10 "/1 -> Motore B/1
  convert/1 -> Motore A/1

== system State_Flow_D/Posizione Vite ==
  Motore vite A : xpcethercatlib/EtherCAT PDO Receive  Priority=2  sig_name=AZ2.Transmit PDO 1.Axis A Actual motor position  sig_offset=272  sig_type=int32  type_size=32  sig_dim=1  device_id=0  sample_time=0.001000
      settings: SourceProductName=Simulink Real-Time  SourceProductBaseCode=XP
  Motore vite B : xpcethercatlib/EtherCAT PDO Receive  Priority=2  sig_name=AZ2.Transmit PDO 2.Axis B Actual motor position  sig_offset=360  sig_type=int32  type_size=32  sig_dim=1  device_id=0  sample_time=0.001000
      settings: SourceProductName=Simulink Real-Time  SourceProductBaseCode=XP
  convert : DataTypeConversion
  "convert 10 " : DataTypeConversion
  Motore A : Outport
  Motore B : Outport  Port=2
  wires:
  Motore vite B/1 -> "convert 10 "/1
  Motore vite A/1 -> convert/1
  "convert 10 "/1 -> Motore B/1
  convert/1 -> Motore A/1

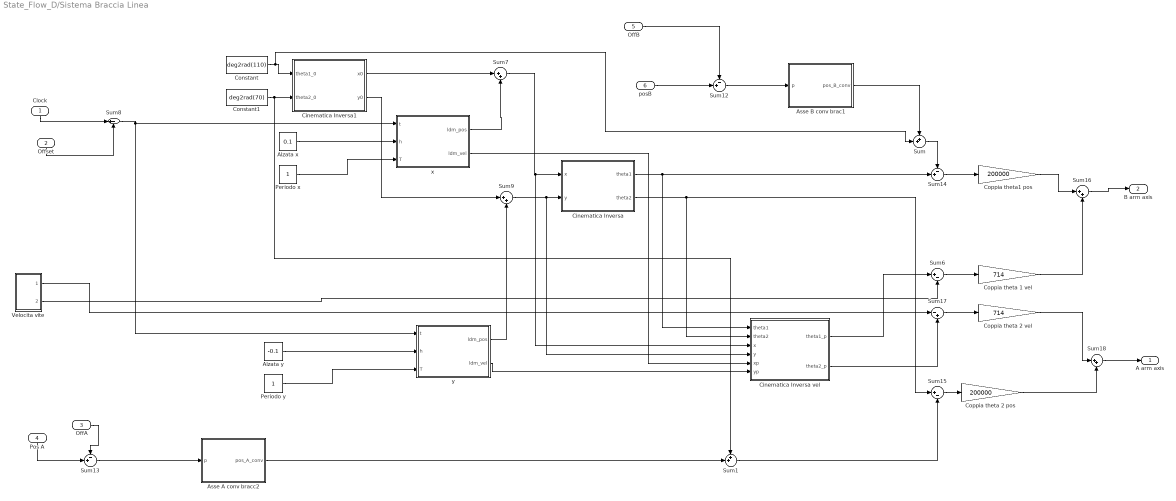
== system State_Flow_D/Sistema Braccia Linea ==
  Clock : Inport
  Offset : Inport  Port=2
  OffA : Inport  Port=3
  Pos A : Inport  Port=4
  OffB : Inport  Port=5
  posB : Inport  Port=6
  Alzata x : Constant  Value=0.1
  Alzata y : Constant  Value=-0.1
  Asse A conv bracc2 : MATLAB Function  TreatAsAtomicUnit=on
  Asse B conv brac1 : MATLAB Function  TreatAsAtomicUnit=on
  Cinematica Inversa : MATLAB Function  TreatAsAtomicUnit=on
  Cinematica Inversa vel : MATLAB Function  TreatAsAtomicUnit=on
  Cinematica Inversa1 : MATLAB Function  TreatAsAtomicUnit=on
  Constant : Constant  Value=deg2rad(110)
  Constant1 : Constant  Value=deg2rad(70)
  Coppia theta 1 vel : Gain  Gain=714
  Coppia theta 2 pos : Gain  Gain=200000
  Coppia theta 2 vel : Gain  Gain=714
  Coppia theta1 pos : Gain  Gain=200000
  Periodo x : Constant
  Periodo y : Constant
  Sum : Sum  Inputs=++|
  Sum1 : Sum  Inputs=++|
  Sum12 : Sum  Inputs=-+|
  Sum13 : Sum  Inputs=-+|
  Sum14 : Sum  Inputs=-+|
  Sum15 : Sum  Inputs=|+-
  Sum{7,9,16,18} (4 alike) : Sum  Inputs=|++
  Sum17 : Sum  Inputs=|-+
  Sum6 : Sum  Inputs=|+-
  Sum8 : Sum  Inputs=|+-
  "Velocita vite " : Subsystem
  x : MATLAB Function  TreatAsAtomicUnit=on
  y : MATLAB Function  TreatAsAtomicUnit=on
  "A arm axis " : Outport
  B arm axis : Outport  Port=2
  wires:
  Sum15/1 -> Coppia theta 2 pos/1
  OffB/1 -> Sum12/1
  x/1(ldm_pos) -> Sum7/2
  posB/1 -> Sum12/2
  y/2(ldm_vel) -> Cinematica Inversa vel/6(yp)
  Cinematica Inversa/2(theta2) -> Cinematica Inversa vel/2(theta2), Sum15/1
  Cinematica Inversa1/2(y0) -> Sum9/1
  Constant1/1 -> Sum1/1, Cinematica Inversa1/2(theta2_0)
  y/1(ldm_pos) -> Sum9/2
  Sum12/1 -> Asse B conv brac1/1(p)
  Clock/1 -> Sum8/1
  Alzata x/1 -> x/2(h)
  Sum7/1 -> Cinematica Inversa vel/3(x), Cinematica Inversa/1(x)
  Constant/1 -> Sum/2, Cinematica Inversa1/1(theta1_0)
  Cinematica Inversa1/1(x0) -> Sum7/1
  Alzata y/1 -> y/2(h)
  Sum6/1 -> Coppia theta 1 vel/1
  Pos A/1 -> Sum13/2
  x/2(ldm_vel) -> Cinematica Inversa vel/5(xp)
  Sum8/1 -> y/1(t), x/1(t)
  Periodo x/1 -> x/3(T)
  Cinematica Inversa vel/2(theta2_p) -> Sum17/2
  Offset/1 -> Sum8/2
  Periodo y/1 -> y/3(T)
  Coppia theta 2 pos/1 -> Sum18/2
  "Velocita vite "/2(Asse B) -> Sum6/2
  Cinematica Inversa vel/1(theta1_p) -> Sum6/1
  OffA/1 -> Sum13/1
  Sum9/1 -> Cinematica Inversa vel/4(y), Cinematica Inversa/2(y)
  Coppia theta1 pos/1 -> Sum16/1
  Cinematica Inversa/1(theta1) -> Sum14/2, Cinematica Inversa vel/1(theta1)
  Sum13/1 -> Asse A conv bracc2/1(p)
  Coppia theta 1 vel/1 -> Sum16/2
  Coppia theta 2 vel/1 -> Sum18/1
  Sum14/1 -> Coppia theta1 pos/1
  Sum17/1 -> Coppia theta 2 vel/1
  Asse B conv brac1/1(pos_B_conv) -> Sum/1
  "Velocita vite "/1(Asse A) -> Sum17/1
  Sum16/1 -> B arm axis/1
  Sum18/1 -> "A arm axis "/1
  Asse A conv bracc2/1(pos_A_conv) -> Sum1/2
  Sum/1 -> Sum14/1
  Sum1/1 -> Sum15/2

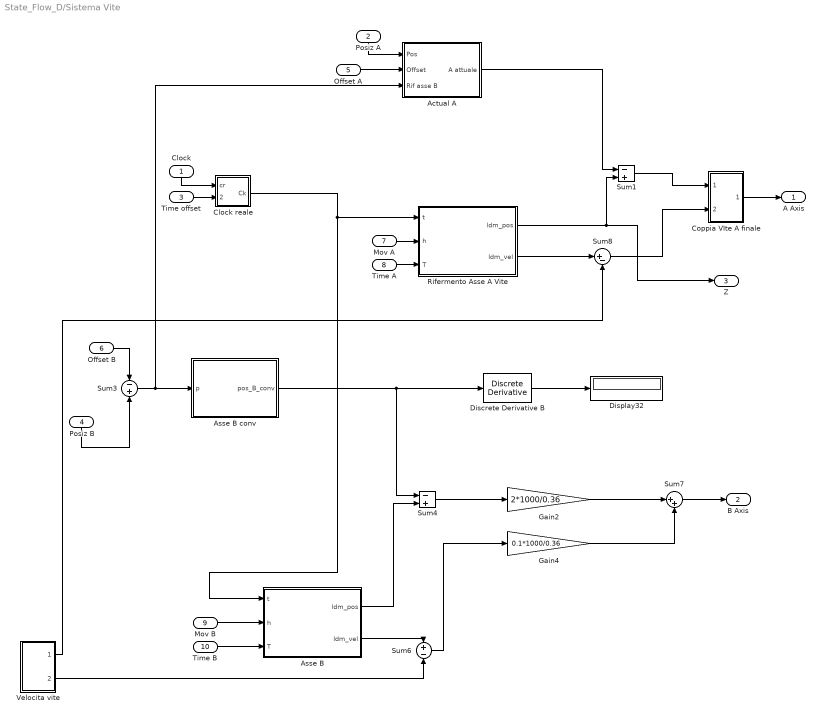
== system State_Flow_D/Sistema Vite ==
  Clock : Inport
  Posiz A : Inport  Port=2
  Time offset : Inport  Port=3
  Posiz B : Inport  Port=4
  Offset A : Inport  Port=5
  Offset B : Inport  Port=6
  Mov A : Inport  Port=7
  Time A : Inport  Port=8
  Mov B : Inport  Port=9
  Time B : Inport  Port=10
  Actual A : Subsystem
  Asse B : MATLAB Function  TreatAsAtomicUnit=on
  Asse B conv : MATLAB Function  TreatAsAtomicUnit=on
  Clock reale : Subsystem
  Coppia VIte A finale : Subsystem
  Discrete Derivative B : simulink/Discrete/Discrete Derivative  gainval=1.0  ICPrevScaledInput=0.0  OutMin=[]  OutMax=[]  OutDataType=fixdt(1, 16)  OutScaling=2^-10  DoSatur=off
  Display32 : Display
  Gain2 : Gain  Gain=2*1000/0.36
  Gain4 : Gain  Gain=0.1*1000/0.36
  Rifermento Asse A Vite : MATLAB Function  TreatAsAtomicUnit=on
  Sum1 : Sum  Inputs=-+
  Sum3 : Sum  Inputs=-|+
  Sum4 : Sum  Inputs=-+
  Sum6 : Sum  Inputs=+|-
  Sum7 : Sum  Inputs=|++
  Sum8 : Sum  Inputs=|+-
  "Velocita vite " : Subsystem
  A Axis : Outport
  B Axis : Outport  Port=2
  Z : Outport  Port=3
  wires:
  Clock/1 -> Clock reale/1(cr)
  Posiz A/1 -> Actual A/1(Pos)
  Offset A/1 -> Actual A/2(Offset)
  Coppia VIte A finale/1(Coppia) -> A Axis/1
  Sum7/1 -> B Axis/1
  Mov A/1 -> Rifermento Asse A Vite/2(h)
  Time A/1 -> Rifermento Asse A Vite/3(T)
  "Velocita vite "/2(Asse B) -> Sum6/2
  Offset B/1 -> Sum3/1
  Asse B conv/1(pos_B_conv) -> Discrete Derivative B/1, Sum4/1
  Asse B/1(ldm_pos) -> Sum4/2
  Sum4/1 -> Gain2/1
  Sum3/1 -> Actual A/3(Rif asse B), Asse B conv/1(p)
  Gain4/1 -> Sum7/2
  Rifermento Asse A Vite/1(ldm_pos) -> Z/1, Sum1/2
  Mov B/1 -> Asse B/2(h)
  Asse B/2(ldm_vel) -> Sum6/1
  "Velocita vite "/1(Asse A) -> Sum8/2
  Gain2/1 -> Sum7/1
  Sum6/1 -> Gain4/1
  Time B/1 -> Asse B/3(T)
  Rifermento Asse A Vite/2(ldm_vel) -> Sum8/1
  Sum1/1 -> Coppia VIte A finale/1(Pos)
  Sum8/1 -> Coppia VIte A finale/2(Vel)
  Actual A/1(A attuale) -> Sum1/1
  Clock reale/1(Ck) -> Asse B/1(t), Rifermento Asse A Vite/1(t)
  Time offset/1 -> Clock reale/2(offset)
  Discrete Derivative B/1 -> Display32/1
  Posiz B/1 -> Sum3/2

== system State_Flow_D/State flow robot/Homing ==
  fc : Inport  OutDataTypeStr=double  PortDimensions=1
  fcA : Inport  Port=2  OutDataTypeStr=double  PortDimensions=1
  fcB : Inport  Port=3  OutDataTypeStr=double  PortDimensions=1
  f : TriggerPort  TriggerType=function-call  VariantControl=Variant  SampleTimeType=periodic  SampleTime=-1
      settings: CopyFcn=Stateflow.SLINSF.SimulinkMan.removeBlockPreDeleteFcn  PreDeleteFcn=Stateflow.SLINSF.SimulinkMan.unsafePredeleteFcn
  MATLAB Function : MATLAB Function  TreatAsAtomicUnit=on
  CA : Outport
  CB : Outport  Port=2
  CH : Outport  Port=3
  wires:
  fc/1 -> MATLAB Function/1(fc)
  fcB/1 -> MATLAB Function/3(fcB)
  fcA/1 -> MATLAB Function/2(fcA)
  MATLAB Function/1(CA) -> CA/1
  MATLAB Function/2(CB) -> CB/1
  MATLAB Function/3(CH) -> CH/1

== system State_Flow_D/Status ==
  Data Type Conversion6 : DataTypeConversion
  Status Word : xpcethercatlib/EtherCAT PDO Receive  Priority=2  sig_name=AZ2.Transmit PDO 4.Axis A Status word  sig_offset=456  sig_type=uint16  type_size=16  sig_dim=1  device_id=0  sample_time=0.001000
      settings: SourceProductName=Simulink Real-Time  SourceProductBaseCode=XP
  Word : Outport
  wires:
  Data Type Conversion6/1 -> Word/1
  Status Word/1 -> Data Type Conversion6/1

== system State_Flow_D/Velocita vite  ==
  EtherCAT PDO Receive14 : xpcethercatlib/EtherCAT PDO Receive  Priority=2  sig_name=AZ1.Transmit PDO 1.Axis A Actual motor velocity  sig_offset=48  sig_type=int32  type_size=32  sig_dim=1  device_id=0  sample_time=0.001000
      settings: SourceProductName=Simulink Real-Time  SourceProductBaseCode=XP
  EtherCAT PDO Receive15 : xpcethercatlib/EtherCAT PDO Receive  Priority=2  sig_name=AZ1.Transmit PDO 2.Axis B Actual motor velocity  sig_offset=136  sig_type=int32  type_size=32  sig_dim=1  device_id=0  sample_time=0.001000
      settings: SourceProductName=Simulink Real-Time  SourceProductBaseCode=XP
  Vel Asse A conv : MATLAB Function  TreatAsAtomicUnit=on
  Vel Asse B conv : MATLAB Function  TreatAsAtomicUnit=on
  Velocity A : DataTypeConversion
  Velocity B : DataTypeConversion
  Asse A : Outport
  Asse B : Outport  Port=2
  wires:
  EtherCAT PDO Receive15/1 -> Velocity B/1
  EtherCAT PDO Receive14/1 -> Velocity A/1
  Vel Asse A conv/1(vel_A_conv) -> Asse A/1
  Velocity B/1 -> Vel Asse B conv/1(p)
  Vel Asse B conv/1(vel_B_conv) -> Asse B/1
  Velocity A/1 -> Vel Asse A conv/1(vA)

== system State_Flow_D/Movimento/Clock reale ==
  cr : Inport
  offset : Inport  Port=2
  Sum2 : Sum  Inputs=-+|
  Ck : Outport
  wires:
  Sum2/1 -> Ck/1
  offset/1 -> Sum2/1
  cr/1 -> Sum2/2

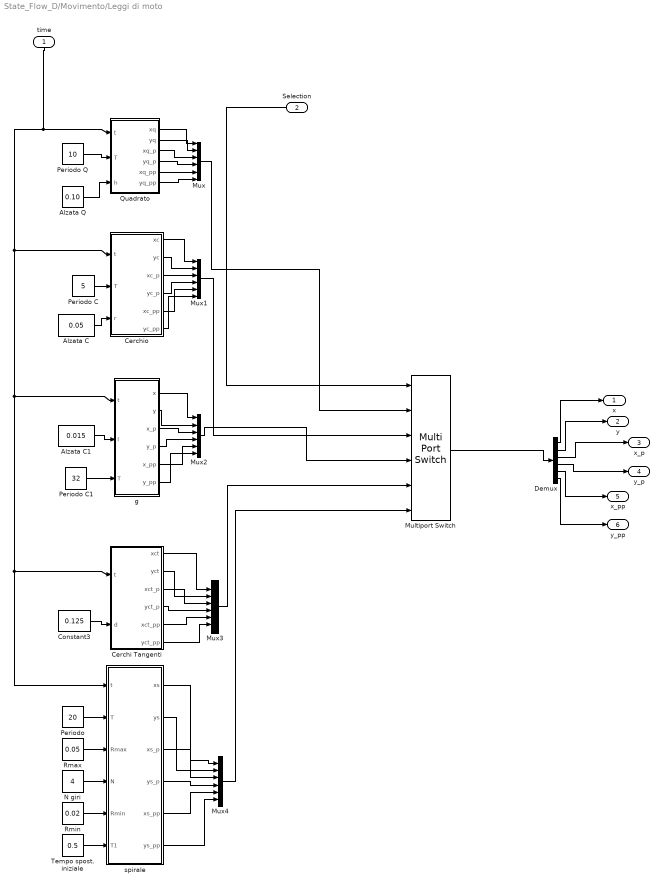
== system State_Flow_D/Movimento/Leggi di moto ==
  time : Inport
  Selection : Inport  Port=2
  Alzata C : Constant  Value=0.05
  Alzata C1 : Constant  Value=0.015
  Alzata Q : Constant  Value=0.10
  Cerchi Tangenti : MATLAB Function  TreatAsAtomicUnit=on
  Cerchio : MATLAB Function  TreatAsAtomicUnit=on
  Constant3 : Constant  Value=0.125
  Demux : Demux  Outputs=6
  Multiport Switch : MultiPortSwitch  Inputs=5
  Mux{,1..4} (5 alike) : Mux  Inputs=6
  N giri : Constant  Value=4
  Periodo : Constant  Value=20
  Periodo C : Constant  Value=5
  Periodo C1 : Constant  Value=32
  Periodo Q : Constant  Value=10
  Quadrato : MATLAB Function  TreatAsAtomicUnit=on
  Rmax : Constant  Value=0.05
  Rmin : Constant  Value=0.02
  Tempo spost. iniziale : Constant  Value=0.5
  g : MATLAB Function  TreatAsAtomicUnit=on
  spirale : MATLAB Function  TreatAsAtomicUnit=on
  x : Outport
  y : Outport  Port=2
  x_p : Outport  Port=3
  y_p : Outport  Port=4
  x_pp : Outport  Port=5
  y_pp : Outport  Port=6
  wires:
  Cerchio/2(yc) -> Mux1/2
  Cerchio/3(xc_p) -> Mux1/3
  Cerchio/4(yc_p) -> Mux1/4
  Cerchio/1(xc) -> Mux1/1
  Mux4/1 -> Multiport Switch/6
  Mux2/1 -> Multiport Switch/4
  spirale/4(ys_p) -> Mux4/4
  Quadrato/2(yq) -> Mux/2
  Quadrato/3(xq_p) -> Mux/3
  Quadrato/4(yq_p) -> Mux/4
  g/1(x) -> Mux2/1
  Demux/2 -> y/1
  Demux/1 -> x/1
  Selection/1 -> Multiport Switch/1
  time/1 -> Quadrato/1(t), Cerchio/1(t), g/1(t), Cerchi Tangenti/1(t), spirale/1(t)
  spirale/3(xs_p) -> Mux4/3
  spirale/2(ys) -> Mux4/2
  g/3(x_p) -> Mux2/3
  g/4(y_p) -> Mux2/4
  Cerchi Tangenti/2(yct) -> Mux3/2
  Cerchi Tangenti/1(xct) -> Mux3/1
  Cerchi Tangenti/4(yct_p) -> Mux3/4
  Cerchi Tangenti/3(xct_p) -> Mux3/3
  Quadrato/1(xq) -> Mux/1
  g/2(y) -> Mux2/2
  spirale/1(xs) -> Mux4/1
  Periodo C/1 -> Cerchio/2(T)
  Periodo Q/1 -> Quadrato/2(T)
  Alzata C/1 -> Cerchio/3(r)
  Alzata Q/1 -> Quadrato/3(h)
  Periodo/1 -> spirale/2(T)
  Constant3/1 -> Cerchi Tangenti/2(d)
  N giri/1 -> spirale/4(N)
  Rmin/1 -> spirale/5(Rmin)
  Tempo spost. iniziale/1 -> spirale/6(T1)
  Alzata C1/1 -> g/2(l)
  Periodo C1/1 -> g/3(T)
  Rmax/1 -> spirale/3(Rmax)
  Multiport Switch/1 -> Demux/1
  Mux3/1 -> Multiport Switch/5
  Mux/1 -> Multiport Switch/2
  Mux1/1 -> Multiport Switch/3
  Demux/3 -> x_p/1
  Demux/4 -> y_p/1
  Cerchio/5(xc_pp) -> Mux1/5
  Cerchio/6(yc_pp) -> Mux1/6
  Demux/5 -> x_pp/1
  Demux/6 -> y_pp/1
  Quadrato/5(xq_pp) -> Mux/5
  Quadrato/6(yq_pp) -> Mux/6
  g/5(x_pp) -> Mux2/5
  g/6(y_pp) -> Mux2/6
  Cerchi Tangenti/5(xct_pp) -> Mux3/5
  Cerchi Tangenti/6(yct_pp) -> Mux3/6
  spirale/5(xs_pp) -> Mux4/5
  spirale/6(ys_pp) -> Mux4/6

== system State_Flow_D/Movimento/Pos iniziali ==
  Cinematica Inversa2 : MATLAB Function  TreatAsAtomicUnit=on
  Constant : Constant  Value=deg2rad(100)
  Constant1 : Constant  Value=deg2rad(80)
  x0 : Outport
  y0 : Outport  Port=2
  wires:
  Cinematica Inversa2/1(x0) -> x0/1
  Cinematica Inversa2/2(y0) -> y0/1
  Constant/1 -> Cinematica Inversa2/1(theta1_0)
  Constant1/1 -> Cinematica Inversa2/2(theta2_0)

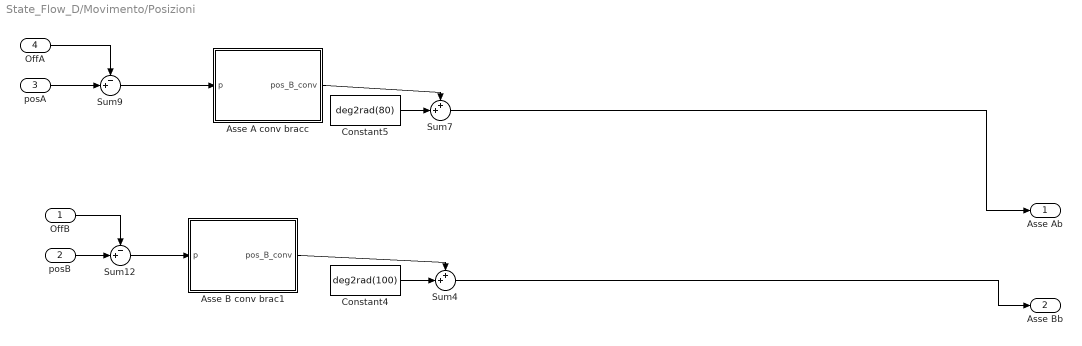
== system State_Flow_D/Movimento/Posizioni ==
  OffB : Inport
  posB : Inport  Port=2
  posA : Inport  Port=3
  OffA : Inport  Port=4
  Asse A conv bracc : MATLAB Function  TreatAsAtomicUnit=on
  Asse B conv brac1 : MATLAB Function  TreatAsAtomicUnit=on
  Constant4 : Constant  Value=deg2rad(100)
  Constant5 : Constant  Value=deg2rad(80)
  Sum12 : Sum  Inputs=-+|
  Sum4 : Sum  Inputs=++|
  Sum7 : Sum  Inputs=++|
  Sum9 : Sum  Inputs=-+|
  Asse Ab : Outport
  Asse Bb : Outport  Port=2
  wires:
  Sum9/1 -> Asse A conv bracc/1(p)
  posB/1 -> Sum12/2
  Sum4/1 -> Asse Bb/1
  OffB/1 -> Sum12/1
  Constant4/1 -> Sum4/2
  Sum7/1 -> Asse Ab/1
  Asse A conv bracc/1(pos_B_conv) -> Sum7/1
  Asse B conv brac1/1(pos_B_conv) -> Sum4/1
  Sum12/1 -> Asse B conv brac1/1(p)
  Constant5/1 -> Sum7/2
  OffA/1 -> Sum9/1
  posA/1 -> Sum9/2

== system State_Flow_D/Movimento/Velocita vite  ==
  EtherCAT PDO Receive14 : xpcethercatlib/EtherCAT PDO Receive  Priority=2  sig_name=AZ1.Transmit PDO 1.Axis A Actual motor velocity  sig_offset=48  sig_type=int32  type_size=32  sig_dim=1  device_id=0  sample_time=0.001000
      settings: SourceProductName=Simulink Real-Time  SourceProductBaseCode=XP
  EtherCAT PDO Receive15 : xpcethercatlib/EtherCAT PDO Receive  Priority=2  sig_name=AZ1.Transmit PDO 2.Axis B Actual motor velocity  sig_offset=136  sig_type=int32  type_size=32  sig_dim=1  device_id=0  sample_time=0.001000
      settings: SourceProductName=Simulink Real-Time  SourceProductBaseCode=XP
  Vel Asse A conv : MATLAB Function  TreatAsAtomicUnit=on
  Vel Asse B conv : MATLAB Function  TreatAsAtomicUnit=on
  Velocity A : DataTypeConversion
  Velocity B : DataTypeConversion
  Asse B : Outport
  Asse A : Outport  Port=2
  wires:
  EtherCAT PDO Receive15/1 -> Velocity B/1
  EtherCAT PDO Receive14/1 -> Velocity A/1
  Vel Asse A conv/1(vel_A_conv) -> Asse A/1
  Velocity B/1 -> Vel Asse B conv/1(p)
  Vel Asse B conv/1(vel_B_conv) -> Asse B/1
  Velocity A/1 -> Vel Asse A conv/1(vA)

== system State_Flow_D/Movimento/Velocita vite 1 ==
  EtherCAT PDO Receive14 : xpcethercatlib/EtherCAT PDO Receive  Priority=2  sig_name=AZ1.Transmit PDO 1.Axis A Actual motor velocity  sig_offset=48  sig_type=int32  type_size=32  sig_dim=1  device_id=0  sample_time=0.001000
      settings: SourceProductName=Simulink Real-Time  SourceProductBaseCode=XP
  EtherCAT PDO Receive15 : xpcethercatlib/EtherCAT PDO Receive  Priority=2  sig_name=AZ1.Transmit PDO 2.Axis B Actual motor velocity  sig_offset=136  sig_type=int32  type_size=32  sig_dim=1  device_id=0  sample_time=0.001000
      settings: SourceProductName=Simulink Real-Time  SourceProductBaseCode=XP
  Vel Asse A conv : MATLAB Function  TreatAsAtomicUnit=on
  Vel Asse B conv : MATLAB Function  TreatAsAtomicUnit=on
  Velocity A : DataTypeConversion
  Velocity B : DataTypeConversion
  Asse B : Outport
  Asse A : Outport  Port=2
  wires:
  EtherCAT PDO Receive15/1 -> Velocity B/1
  EtherCAT PDO Receive14/1 -> Velocity A/1
  Vel Asse A conv/1(vel_A_conv) -> Asse A/1
  Velocity B/1 -> Vel Asse B conv/1(p)
  Vel Asse B conv/1(vel_B_conv) -> Asse B/1
  Velocity A/1 -> Vel Asse A conv/1(vA)

== system State_Flow_D/Movimento Braccia/Clock reale ==
  cr : Inport
  offset : Inport  Port=2
  Sum2 : Sum  Inputs=-+|
  Ck : Outport
  wires:
  Sum2/1 -> Ck/1
  offset/1 -> Sum2/1
  cr/1 -> Sum2/2

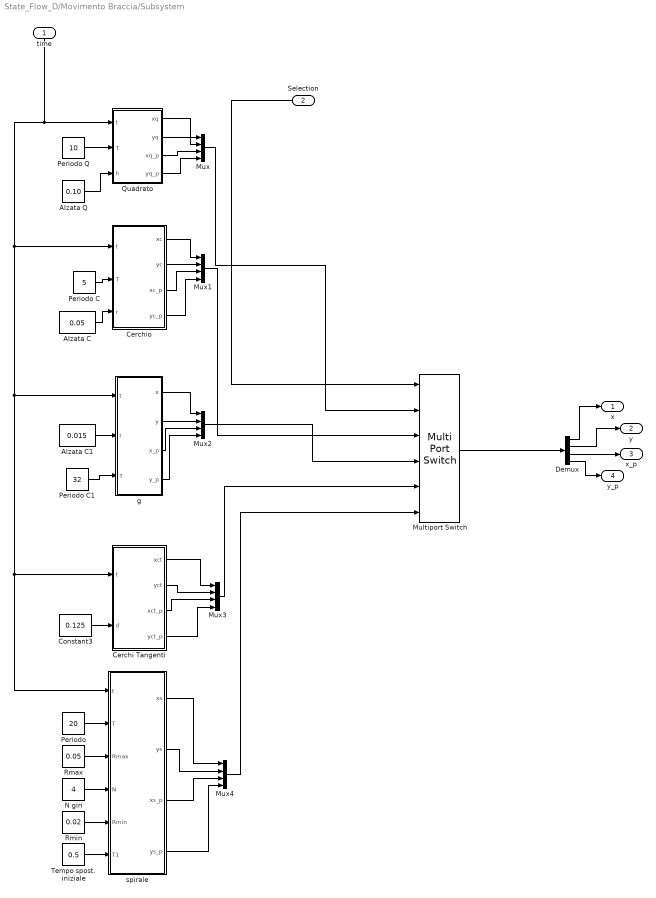
== system State_Flow_D/Movimento Braccia/Subsystem ==
  time : Inport
  Selection : Inport  Port=2
  Alzata C : Constant  Value=0.05
  Alzata C1 : Constant  Value=0.015
  Alzata Q : Constant  Value=0.10
  Cerchi Tangenti : MATLAB Function  TreatAsAtomicUnit=on
  Cerchio : MATLAB Function  TreatAsAtomicUnit=on
  Constant3 : Constant  Value=0.125
  Demux : Demux
  Multiport Switch : MultiPortSwitch  Inputs=5
  Mux{,1..4} (5 alike) : Mux
  N giri : Constant  Value=4
  Periodo : Constant  Value=20
  Periodo C : Constant  Value=5
  Periodo C1 : Constant  Value=32
  Periodo Q : Constant  Value=10
  Quadrato : MATLAB Function  TreatAsAtomicUnit=on
  Rmax : Constant  Value=0.05
  Rmin : Constant  Value=0.02
  Tempo spost. iniziale : Constant  Value=0.5
  g : MATLAB Function  TreatAsAtomicUnit=on
  spirale : MATLAB Function  TreatAsAtomicUnit=on
  x : Outport
  y : Outport  Port=2
  x_p : Outport  Port=3
  y_p : Outport  Port=4
  wires:
  Cerchio/2(yc) -> Mux1/2
  Cerchio/3(xc_p) -> Mux1/3
  Cerchio/4(yc_p) -> Mux1/4
  Cerchio/1(xc) -> Mux1/1
  Mux4/1 -> Multiport Switch/6
  Mux2/1 -> Multiport Switch/4
  spirale/4(ys_p) -> Mux4/4
  Quadrato/2(yq) -> Mux/2
  Quadrato/3(xq_p) -> Mux/3
  Quadrato/4(yq_p) -> Mux/4
  g/1(x) -> Mux2/1
  Demux/2 -> y/1
  Demux/1 -> x/1
  Selection/1 -> Multiport Switch/1
  time/1 -> Quadrato/1(t), Cerchio/1(t), g/1(t), Cerchi Tangenti/1(t), spirale/1(t)
  spirale/3(xs_p) -> Mux4/3
  spirale/2(ys) -> Mux4/2
  g/3(x_p) -> Mux2/3
  g/4(y_p) -> Mux2/4
  Cerchi Tangenti/2(yct) -> Mux3/2
  Cerchi Tangenti/1(xct) -> Mux3/1
  Cerchi Tangenti/4(yct_p) -> Mux3/4
  Cerchi Tangenti/3(xct_p) -> Mux3/3
  Quadrato/1(xq) -> Mux/1
  g/2(y) -> Mux2/2
  spirale/1(xs) -> Mux4/1
  Periodo C/1 -> Cerchio/2(T)
  Periodo Q/1 -> Quadrato/2(T)
  Alzata C/1 -> Cerchio/3(r)
  Alzata Q/1 -> Quadrato/3(h)
  Periodo/1 -> spirale/2(T)
  Constant3/1 -> Cerchi Tangenti/2(d)
  N giri/1 -> spirale/4(N)
  Rmin/1 -> spirale/5(Rmin)
  Tempo spost. iniziale/1 -> spirale/6(T1)
  Alzata C1/1 -> g/2(l)
  Periodo C1/1 -> g/3(T)
  Rmax/1 -> spirale/3(Rmax)
  Multiport Switch/1 -> Demux/1
  Mux3/1 -> Multiport Switch/5
  Mux/1 -> Multiport Switch/2
  Mux1/1 -> Multiport Switch/3
  Demux/3 -> x_p/1
  Demux/4 -> y_p/1

== system State_Flow_D/Movimento Braccia/Velocita vite  ==
  EtherCAT PDO Receive14 : xpcethercatlib/EtherCAT PDO Receive  Priority=2  sig_name=AZ1.Transmit PDO 1.Axis A Actual motor velocity  sig_offset=48  sig_type=int32  type_size=32  sig_dim=1  device_id=0  sample_time=0.001000
      settings: SourceProductName=Simulink Real-Time  SourceProductBaseCode=XP
  EtherCAT PDO Receive15 : xpcethercatlib/EtherCAT PDO Receive  Priority=2  sig_name=AZ1.Transmit PDO 2.Axis B Actual motor velocity  sig_offset=136  sig_type=int32  type_size=32  sig_dim=1  device_id=0  sample_time=0.001000
      settings: SourceProductName=Simulink Real-Time  SourceProductBaseCode=XP
  Vel Asse A conv : MATLAB Function  TreatAsAtomicUnit=on
  Vel Asse B conv : MATLAB Function  TreatAsAtomicUnit=on
  Velocity A : DataTypeConversion
  Velocity B : DataTypeConversion
  Asse B : Outport
  Asse A : Outport  Port=2
  wires:
  EtherCAT PDO Receive15/1 -> Velocity B/1
  EtherCAT PDO Receive14/1 -> Velocity A/1
  Vel Asse A conv/1(vel_A_conv) -> Asse A/1
  Velocity B/1 -> Vel Asse B conv/1(p)
  Vel Asse B conv/1(vel_B_conv) -> Asse B/1
  Velocity A/1 -> Vel Asse A conv/1(vA)

== system State_Flow_D/Out Asse A Braccia/Fungo ==
  In1 : Inport
  Constant : Constant  Value=0
  Data Type Conversion14 : DataTypeConversion
  Display10 : Display
  EtherCAT PDO Receive9 : xpcethercatlib/EtherCAT PDO Receive  Priority=2  sig_name=Beckoff.Channel 1.Input  sig_offset=0  sig_type=boolean  type_size=1  sig_dim=1  device_id=0  sample_time=0.001000
      settings: SourceProductName=Simulink Real-Time  SourceProductBaseCode=XP
  MATLAB Function : MATLAB Function  TreatAsAtomicUnit=on
  Memory : Memory
  Switch1 : Switch  Criteria=u2 ~= 0  Threshold=2
  Out1 : Outport
  wires:
  EtherCAT PDO Receive9/1 -> Data Type Conversion14/1
  Data Type Conversion14/1 -> MATLAB Function/2(old), Display10/1
  MATLAB Function/1(y) -> Memory/1
  In1/1 -> Switch1/3
  Memory/1 -> Switch1/2, MATLAB Function/1(now)
  Constant/1 -> Switch1/1
  Switch1/1 -> Out1/1

== system State_Flow_D/Out Asse B Braccia/Fungo ==
  In1 : Inport
  Constant : Constant  Value=0
  Data Type Conversion14 : DataTypeConversion
  Display10 : Display
  EtherCAT PDO Receive9 : xpcethercatlib/EtherCAT PDO Receive  Priority=2  sig_name=Beckoff.Channel 1.Input  sig_offset=0  sig_type=boolean  type_size=1  sig_dim=1  device_id=0  sample_time=0.001000
      settings: SourceProductName=Simulink Real-Time  SourceProductBaseCode=XP
  MATLAB Function : MATLAB Function  TreatAsAtomicUnit=on
  Memory : Memory
  Switch1 : Switch  Criteria=u2 ~= 0  Threshold=2
  Out1 : Outport
  wires:
  EtherCAT PDO Receive9/1 -> Data Type Conversion14/1
  Data Type Conversion14/1 -> MATLAB Function/2(old), Display10/1
  MATLAB Function/1(y) -> Memory/1
  In1/1 -> Switch1/3
  Memory/1 -> Switch1/2, MATLAB Function/1(now)
  Constant/1 -> Switch1/1
  Switch1/1 -> Out1/1

== system State_Flow_D/Out asse A Vite/Fungo ==
  In1 : Inport
  Constant : Constant  Value=0
  Data Type Conversion14 : DataTypeConversion
  Display10 : Display
  EtherCAT PDO Receive9 : xpcethercatlib/EtherCAT PDO Receive  Priority=2  sig_name=Beckoff.Channel 1.Input  sig_offset=0  sig_type=boolean  type_size=1  sig_dim=1  device_id=0  sample_time=0.001000
      settings: SourceProductName=Simulink Real-Time  SourceProductBaseCode=XP
  MATLAB Function : MATLAB Function  TreatAsAtomicUnit=on
  Memory : Memory
  Switch1 : Switch  Criteria=u2 ~= 0  Threshold=2
  Out1 : Outport
  wires:
  EtherCAT PDO Receive9/1 -> Data Type Conversion14/1
  Data Type Conversion14/1 -> MATLAB Function/2(old), Display10/1
  MATLAB Function/1(y) -> Memory/1
  In1/1 -> Switch1/3
  Memory/1 -> Switch1/2, MATLAB Function/1(now)
  Constant/1 -> Switch1/1
  Switch1/1 -> Out1/1
